simulink model "Prak1Aufg2Simulink"  (Simulink 7.7)
settings: Solver=ode45  StartTime=0.0  StopTime=100.0  RelTol=1e-3
settings Model: Creator=hexren  LastModifiedBy=hexren

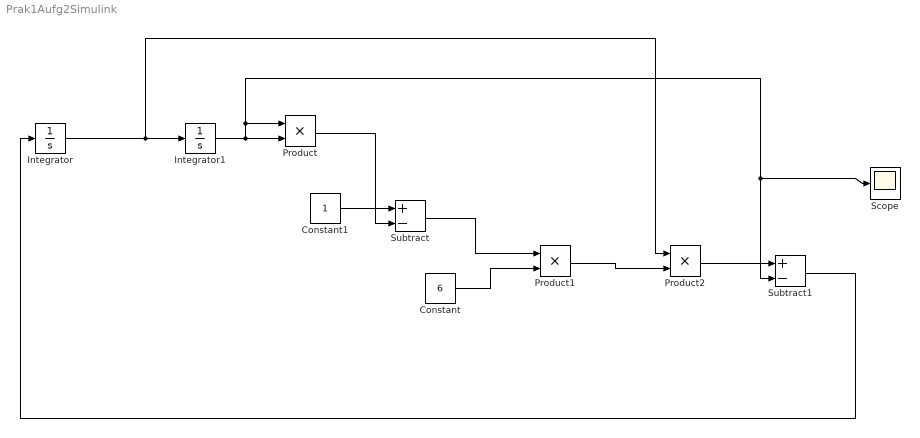
== system Prak1Aufg2Simulink ==
  Constant : Constant  Value=6
  Constant1 : Constant
  Integrator : Integrator  InitialCondition=1
  Integrator1 : Integrator
  Product : Product  RndMeth=Zero
  Product1 : Product  RndMeth=Zero
  Product2 : Product  RndMeth=Zero
  Scope : Scope
  Subtract : Sum  Inputs=+-
  Subtract1 : Sum  Inputs=+-
  wires:
  Integrator/1 -> Integrator1/1, Product2/1
  Constant1/1 -> Subtract/1
  Integrator1/1 -> Product/2, Product/1, Subtract1/2, Scope/1
  Product/1 -> Subtract/2
  Subtract/1 -> Product1/1
  Constant/1 -> Product1/2
  Product1/1 -> Product2/2
  Product2/1 -> Subtract1/1
  Subtract1/1 -> Integrator/1
